simulink model "MPCSimulation"  (Simulink 9.2)
settings: Solver=ode45  StartTime=0.0  StopTime=100  RelTol=1e-3  EnableMultiTasking=on
values from neighbouring files (symbols this model uses):
  A = plant.A    [MPCController.m]    (also in SlowMPCController.m = Plant.A; Untitled.m = [0,0,0;0,0,0;-1,1,0]; setupsimulation.m = [0,0;1,0])
  B = plant.B    [MPCController.m]    (also in SlowMPCController.m = Plant.B; Untitled.m = [0;1;0]; setupsimulation.m = [1;0])
  C = plant.C    [MPCController.m]    (also in SlowMPCController.m = Plant.C; Untitled.m = [0,0,1]; setupsimulation.m = [0,1])
undefined symbols (not defined in the file or in its folder): MPCController
settings Model: Creator=johanl  LastModifiedBy=HP
settings OptimizationCC: ExpressionDepthLimit=2147483647
settings DebuggingCC: SolverPrmCheckMsg=warning  LibraryContextMissingDiagnostic=none
settings GRTTargetCC: CombineOutputUpdateFcns=on  GRTInterface=off

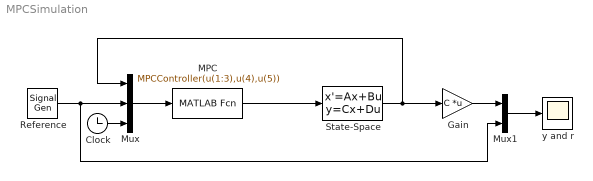
== system MPCSimulation ==
  Clock : Clock
      settings: Decimation=100
  Gain : Gain  Gain=C  Multiplication=Matrix(K*u)
  MPC : MATLABFcn  MATLABFcn=MPCController(u(1:3),u(4),u(5))
  Mux : Mux  Inputs=3
  Mux1 : Mux  Inputs=2
  Reference : SignalGenerator  WaveForm=square  Frequency=0.05
  State-Space : StateSpace  A=A  B=B  C=eye(3)  D=zeros(3,1)  InitialCondition=[0,0,0]
  y and r : Scope
  wires:
  Clock/1 -> Mux/3
  State-Space/1 -> Gain/1, Mux/1
  MPC/1 -> State-Space/1
  Gain/1 -> Mux1/1
  Mux1/1 -> y and r/1
  Mux/1 -> MPC/1
  Reference/1 -> Mux/2, Mux1/2
